simulink model "Simulator_3D2"  (R2018a)
settings: Solver=ode4  StartTime=0.0  StopTime=60  FixedStep=T  RelTol=1e-3
undefined symbols (not defined in the file): A_w, A_w2, epsilon_w, epsilon_w2, k_w, k_w2, Lc_0, omega_w, omega_w2, T, w_dir, w_dir2, zu_bar
libraries: vrlib x132
(part 6 of 6)

== system Simulator_3D2/Subsystem/5 static wave points7/Subsystem15/Subsystem ==
  note: Aw.Sin
  t : Inport
  x : Inport  Port=2
  Constant : Constant  Value=epsilon_w
  Gain : Gain  Gain=omega_w
  Gain1 : Gain  Gain=k_w
  Gain2 : Gain  Gain=A_w
  Gain5 : Gain  Gain=A_w*k_w
  Sum : Sum  Inputs=++-
  Trigonometric Function1 : Trigonometry  Operator=sincos
  Trigonometric Function2 : Trigonometry  Operator=atan
  direction : Gain  Gain=w_dir
  zeta(x,t) : Outport
  theta : Outport  Port=2
  wires:
  Trigonometric Function2/1 -> theta/1
  Gain5/1 -> Trigonometric Function2/1
  Trigonometric Function1/2 -> Gain5/1
  Gain/1 -> Sum/2
  Gain2/1 -> zeta(x,t)/1  "zeta(x,t)"
  Constant/1 -> Sum/1
  t/1 -> direction/1
  Gain1/1 -> Sum/3
  Trigonometric Function1/1 -> Gain2/1
  x/1 -> Gain1/1
  direction/1 -> Gain/1
  Sum/1 -> Trigonometric Function1/1

== system Simulator_3D2/Subsystem/5 static wave points7/Subsystem15/Subsystem1 ==
  note: Aw.Sin
  t : Inport
  x : Inport  Port=2
  Constant : Constant  Value=epsilon_w2
  Gain : Gain  Gain=omega_w2
  Gain1 : Gain  Gain=k_w2
  Gain2 : Gain  Gain=A_w2
  Gain5 : Gain  Gain=A_w2*k_w2
  Sum : Sum  Inputs=++-
  Trigonometric Function : Trigonometry  Operator=sincos
  Trigonometric Function1 : Trigonometry  Operator=atan
  direction : Gain  Gain=w_dir2
  zeta(x,t) : Outport
  theta : Outport  Port=2
  wires:
  Trigonometric Function/2 -> Gain5/1
  Trigonometric Function1/1 -> theta/1
  Gain5/1 -> Trigonometric Function1/1
  Sum/1 -> Trigonometric Function/1
  direction/1 -> Gain/1
  x/1 -> Gain1/1
  Trigonometric Function/1 -> Gain2/1
  Gain1/1 -> Sum/3
  t/1 -> direction/1
  Constant/1 -> Sum/1
  Gain2/1 -> zeta(x,t)/1  "zeta(x,t)"
  Gain/1 -> Sum/2

== system Simulator_3D2/Subsystem/5 static wave points7/Subsystem16/Subsystem ==
  note: Aw.Sin
  t : Inport
  x : Inport  Port=2
  Constant : Constant  Value=epsilon_w
  Gain : Gain  Gain=omega_w
  Gain1 : Gain  Gain=k_w
  Gain2 : Gain  Gain=A_w
  Gain5 : Gain  Gain=A_w*k_w
  Sum : Sum  Inputs=++-
  Trigonometric Function1 : Trigonometry  Operator=sincos
  Trigonometric Function2 : Trigonometry  Operator=atan
  direction : Gain  Gain=w_dir
  zeta(x,t) : Outport
  theta : Outport  Port=2
  wires:
  Sum/1 -> Trigonometric Function1/1
  direction/1 -> Gain/1
  x/1 -> Gain1/1
  Trigonometric Function1/1 -> Gain2/1
  Gain1/1 -> Sum/3
  t/1 -> direction/1
  Constant/1 -> Sum/1
  Gain2/1 -> zeta(x,t)/1  "zeta(x,t)"
  Gain/1 -> Sum/2
  Trigonometric Function1/2 -> Gain5/1
  Gain5/1 -> Trigonometric Function2/1
  Trigonometric Function2/1 -> theta/1

== system Simulator_3D2/Subsystem/5 static wave points7/Subsystem16/Subsystem1 ==
  note: Aw.Sin
  t : Inport
  x : Inport  Port=2
  Constant : Constant  Value=epsilon_w2
  Gain : Gain  Gain=omega_w2
  Gain1 : Gain  Gain=k_w2
  Gain2 : Gain  Gain=A_w2
  Gain5 : Gain  Gain=A_w2*k_w2
  Sum : Sum  Inputs=++-
  Trigonometric Function : Trigonometry  Operator=sincos
  Trigonometric Function1 : Trigonometry  Operator=atan
  direction : Gain  Gain=w_dir2
  zeta(x,t) : Outport
  theta : Outport  Port=2
  wires:
  Gain/1 -> Sum/2
  Gain2/1 -> zeta(x,t)/1  "zeta(x,t)"
  Constant/1 -> Sum/1
  t/1 -> direction/1
  Gain1/1 -> Sum/3
  Trigonometric Function/1 -> Gain2/1
  x/1 -> Gain1/1
  direction/1 -> Gain/1
  Sum/1 -> Trigonometric Function/1
  Gain5/1 -> Trigonometric Function1/1
  Trigonometric Function1/1 -> theta/1
  Trigonometric Function/2 -> Gain5/1

== system Simulator_3D2/Subsystem/followers/Subsystem1/Subsystem ==
  note: Aw.Sin
  t : Inport
  x : Inport  Port=2
  Constant : Constant  Value=epsilon_w
  Gain : Gain  Gain=omega_w
  Gain1 : Gain  Gain=k_w
  Gain2 : Gain  Gain=A_w
  Gain5 : Gain  Gain=A_w*k_w
  Sum : Sum  Inputs=++-
  Trigonometric Function1 : Trigonometry  Operator=sincos
  Trigonometric Function2 : Trigonometry  Operator=atan
  direction : Gain  Gain=w_dir
  zeta(x,t) : Outport
  theta : Outport  Port=2
  wires:
  Trigonometric Function2/1 -> theta/1
  Gain5/1 -> Trigonometric Function2/1
  Trigonometric Function1/2 -> Gain5/1
  Gain/1 -> Sum/2
  Gain2/1 -> zeta(x,t)/1  "zeta(x,t)"
  Constant/1 -> Sum/1
  t/1 -> direction/1
  Gain1/1 -> Sum/3
  Trigonometric Function1/1 -> Gain2/1
  x/1 -> Gain1/1
  direction/1 -> Gain/1
  Sum/1 -> Trigonometric Function1/1

== system Simulator_3D2/Subsystem/followers/Subsystem1/Subsystem1 ==
  note: Aw.Sin
  t : Inport
  x : Inport  Port=2
  Constant : Constant  Value=epsilon_w2
  Gain : Gain  Gain=omega_w2
  Gain1 : Gain  Gain=k_w2
  Gain2 : Gain  Gain=A_w2
  Gain5 : Gain  Gain=A_w2*k_w2
  Sum : Sum  Inputs=++-
  Trigonometric Function : Trigonometry  Operator=sincos
  Trigonometric Function1 : Trigonometry  Operator=atan
  direction : Gain  Gain=w_dir2
  zeta(x,t) : Outport
  theta : Outport  Port=2
  wires:
  Trigonometric Function/2 -> Gain5/1
  Trigonometric Function1/1 -> theta/1
  Gain5/1 -> Trigonometric Function1/1
  Sum/1 -> Trigonometric Function/1
  direction/1 -> Gain/1
  x/1 -> Gain1/1
  Trigonometric Function/1 -> Gain2/1
  Gain1/1 -> Sum/3
  t/1 -> direction/1
  Constant/1 -> Sum/1
  Gain2/1 -> zeta(x,t)/1  "zeta(x,t)"
  Gain/1 -> Sum/2

== system Simulator_3D2/Subsystem/followers/Subsystem2/Subsystem ==
  note: Aw.Sin
  t : Inport
  x : Inport  Port=2
  Constant : Constant  Value=epsilon_w
  Gain : Gain  Gain=omega_w
  Gain1 : Gain  Gain=k_w
  Gain2 : Gain  Gain=A_w
  Gain5 : Gain  Gain=A_w*k_w
  Sum : Sum  Inputs=++-
  Trigonometric Function1 : Trigonometry  Operator=sincos
  Trigonometric Function2 : Trigonometry  Operator=atan
  direction : Gain  Gain=w_dir
  zeta(x,t) : Outport
  theta : Outport  Port=2
  wires:
  Sum/1 -> Trigonometric Function1/1
  direction/1 -> Gain/1
  x/1 -> Gain1/1
  Trigonometric Function1/1 -> Gain2/1
  Gain1/1 -> Sum/3
  t/1 -> direction/1
  Constant/1 -> Sum/1
  Gain2/1 -> zeta(x,t)/1  "zeta(x,t)"
  Gain/1 -> Sum/2
  Trigonometric Function1/2 -> Gain5/1
  Gain5/1 -> Trigonometric Function2/1
  Trigonometric Function2/1 -> theta/1

== system Simulator_3D2/Subsystem/followers/Subsystem2/Subsystem1 ==
  note: Aw.Sin
  t : Inport
  x : Inport  Port=2
  Constant : Constant  Value=epsilon_w2
  Gain : Gain  Gain=omega_w2
  Gain1 : Gain  Gain=k_w2
  Gain2 : Gain  Gain=A_w2
  Gain5 : Gain  Gain=A_w2*k_w2
  Sum : Sum  Inputs=++-
  Trigonometric Function : Trigonometry  Operator=sincos
  Trigonometric Function1 : Trigonometry  Operator=atan
  direction : Gain  Gain=w_dir2
  zeta(x,t) : Outport
  theta : Outport  Port=2
  wires:
  Gain/1 -> Sum/2
  Gain2/1 -> zeta(x,t)/1  "zeta(x,t)"
  Constant/1 -> Sum/1
  t/1 -> direction/1
  Gain1/1 -> Sum/3
  Trigonometric Function/1 -> Gain2/1
  x/1 -> Gain1/1
  direction/1 -> Gain/1
  Sum/1 -> Trigonometric Function/1
  Gain5/1 -> Trigonometric Function1/1
  Trigonometric Function1/1 -> theta/1
  Trigonometric Function/2 -> Gain5/1

== system Simulator_3D2/Subsystem/followers/Subsystem3/Subsystem ==
  note: Aw.Sin
  t : Inport
  x : Inport  Port=2
  Constant : Constant  Value=epsilon_w
  Gain : Gain  Gain=omega_w
  Gain1 : Gain  Gain=k_w
  Gain2 : Gain  Gain=A_w
  Gain5 : Gain  Gain=A_w*k_w
  Sum : Sum  Inputs=++-
  Trigonometric Function1 : Trigonometry  Operator=sincos
  Trigonometric Function2 : Trigonometry  Operator=atan
  direction : Gain  Gain=w_dir
  zeta(x,t) : Outport
  theta : Outport  Port=2
  wires:
  Sum/1 -> Trigonometric Function1/1
  direction/1 -> Gain/1
  x/1 -> Gain1/1
  Trigonometric Function1/1 -> Gain2/1
  Gain1/1 -> Sum/3
  t/1 -> direction/1
  Constant/1 -> Sum/1
  Gain2/1 -> zeta(x,t)/1  "zeta(x,t)"
  Gain/1 -> Sum/2
  Trigonometric Function1/2 -> Gain5/1
  Gain5/1 -> Trigonometric Function2/1
  Trigonometric Function2/1 -> theta/1

== system Simulator_3D2/Subsystem/followers/Subsystem3/Subsystem1 ==
  note: Aw.Sin
  t : Inport
  x : Inport  Port=2
  Constant : Constant  Value=epsilon_w2
  Gain : Gain  Gain=omega_w2
  Gain1 : Gain  Gain=k_w2
  Gain2 : Gain  Gain=A_w2
  Gain5 : Gain  Gain=A_w2*k_w2
  Sum : Sum  Inputs=++-
  Trigonometric Function : Trigonometry  Operator=sincos
  Trigonometric Function1 : Trigonometry  Operator=atan
  direction : Gain  Gain=w_dir2
  zeta(x,t) : Outport
  theta : Outport  Port=2
  wires:
  Gain/1 -> Sum/2
  Gain2/1 -> zeta(x,t)/1  "zeta(x,t)"
  Constant/1 -> Sum/1
  t/1 -> direction/1
  Gain1/1 -> Sum/3
  Trigonometric Function/1 -> Gain2/1
  x/1 -> Gain1/1
  direction/1 -> Gain/1
  Sum/1 -> Trigonometric Function/1
  Gain5/1 -> Trigonometric Function1/1
  Trigonometric Function1/1 -> theta/1
  Trigonometric Function/2 -> Gain5/1

== system Simulator_3D2/Subsystem/followers/Subsystem4/Subsystem ==
  note: Aw.Sin
  t : Inport
  x : Inport  Port=2
  Constant : Constant  Value=epsilon_w
  Gain : Gain  Gain=omega_w
  Gain1 : Gain  Gain=k_w
  Gain2 : Gain  Gain=A_w
  Gain5 : Gain  Gain=A_w*k_w
  Sum : Sum  Inputs=++-
  Trigonometric Function1 : Trigonometry  Operator=sincos
  Trigonometric Function2 : Trigonometry  Operator=atan
  direction : Gain  Gain=w_dir
  zeta(x,t) : Outport
  theta : Outport  Port=2
  wires:
  Trigonometric Function2/1 -> theta/1
  Gain5/1 -> Trigonometric Function2/1
  Trigonometric Function1/2 -> Gain5/1
  Gain/1 -> Sum/2
  Gain2/1 -> zeta(x,t)/1  "zeta(x,t)"
  Constant/1 -> Sum/1
  t/1 -> direction/1
  Gain1/1 -> Sum/3
  Trigonometric Function1/1 -> Gain2/1
  x/1 -> Gain1/1
  direction/1 -> Gain/1
  Sum/1 -> Trigonometric Function1/1

== system Simulator_3D2/Subsystem/followers/Subsystem4/Subsystem1 ==
  note: Aw.Sin
  t : Inport
  x : Inport  Port=2
  Constant : Constant  Value=epsilon_w2
  Gain : Gain  Gain=omega_w2
  Gain1 : Gain  Gain=k_w2
  Gain2 : Gain  Gain=A_w2
  Gain5 : Gain  Gain=A_w2*k_w2
  Sum : Sum  Inputs=++-
  Trigonometric Function : Trigonometry  Operator=sincos
  Trigonometric Function1 : Trigonometry  Operator=atan
  direction : Gain  Gain=w_dir2
  zeta(x,t) : Outport
  theta : Outport  Port=2
  wires:
  Trigonometric Function/2 -> Gain5/1
  Trigonometric Function1/1 -> theta/1
  Gain5/1 -> Trigonometric Function1/1
  Sum/1 -> Trigonometric Function/1
  direction/1 -> Gain/1
  x/1 -> Gain1/1
  Trigonometric Function/1 -> Gain2/1
  Gain1/1 -> Sum/3
  t/1 -> direction/1
  Constant/1 -> Sum/1
  Gain2/1 -> zeta(x,t)/1  "zeta(x,t)"
  Gain/1 -> Sum/2

== system Simulator_3D2/Subsystem/followers/Subsystem5/Subsystem ==
  note: Aw.Sin
  t : Inport
  x : Inport  Port=2
  Constant : Constant  Value=epsilon_w
  Gain : Gain  Gain=omega_w
  Gain1 : Gain  Gain=k_w
  Gain2 : Gain  Gain=A_w
  Gain5 : Gain  Gain=A_w*k_w
  Sum : Sum  Inputs=++-
  Trigonometric Function1 : Trigonometry  Operator=sincos
  Trigonometric Function2 : Trigonometry  Operator=atan
  direction : Gain  Gain=w_dir
  zeta(x,t) : Outport
  theta : Outport  Port=2
  wires:
  Sum/1 -> Trigonometric Function1/1
  direction/1 -> Gain/1
  x/1 -> Gain1/1
  Trigonometric Function1/1 -> Gain2/1
  Gain1/1 -> Sum/3
  t/1 -> direction/1
  Constant/1 -> Sum/1
  Gain2/1 -> zeta(x,t)/1  "zeta(x,t)"
  Gain/1 -> Sum/2
  Trigonometric Function1/2 -> Gain5/1
  Gain5/1 -> Trigonometric Function2/1
  Trigonometric Function2/1 -> theta/1

== system Simulator_3D2/Subsystem/followers/Subsystem5/Subsystem1 ==
  note: Aw.Sin
  t : Inport
  x : Inport  Port=2
  Constant : Constant  Value=epsilon_w2
  Gain : Gain  Gain=omega_w2
  Gain1 : Gain  Gain=k_w2
  Gain2 : Gain  Gain=A_w2
  Gain5 : Gain  Gain=A_w2*k_w2
  Sum : Sum  Inputs=++-
  Trigonometric Function : Trigonometry  Operator=sincos
  Trigonometric Function1 : Trigonometry  Operator=atan
  direction : Gain  Gain=w_dir2
  zeta(x,t) : Outport
  theta : Outport  Port=2
  wires:
  Gain/1 -> Sum/2
  Gain2/1 -> zeta(x,t)/1  "zeta(x,t)"
  Constant/1 -> Sum/1
  t/1 -> direction/1
  Gain1/1 -> Sum/3
  Trigonometric Function/1 -> Gain2/1
  x/1 -> Gain1/1
  direction/1 -> Gain/1
  Sum/1 -> Trigonometric Function/1
  Gain5/1 -> Trigonometric Function1/1
  Trigonometric Function1/1 -> theta/1
  Trigonometric Function/2 -> Gain5/1

== system Simulator_3D2/Subsystem/followers/Subsystem6/Subsystem ==
  note: Aw.Sin
  t : Inport
  x : Inport  Port=2
  Constant : Constant  Value=epsilon_w
  Gain : Gain  Gain=omega_w
  Gain1 : Gain  Gain=k_w
  Gain2 : Gain  Gain=A_w
  Gain5 : Gain  Gain=A_w*k_w
  Sum : Sum  Inputs=++-
  Trigonometric Function1 : Trigonometry  Operator=sincos
  Trigonometric Function2 : Trigonometry  Operator=atan
  direction : Gain  Gain=w_dir
  zeta(x,t) : Outport
  theta : Outport  Port=2
  wires:
  Trigonometric Function2/1 -> theta/1
  Gain5/1 -> Trigonometric Function2/1
  Trigonometric Function1/2 -> Gain5/1
  Gain/1 -> Sum/2
  Gain2/1 -> zeta(x,t)/1  "zeta(x,t)"
  Constant/1 -> Sum/1
  t/1 -> direction/1
  Gain1/1 -> Sum/3
  Trigonometric Function1/1 -> Gain2/1
  x/1 -> Gain1/1
  direction/1 -> Gain/1
  Sum/1 -> Trigonometric Function1/1

== system Simulator_3D2/Subsystem/followers/Subsystem6/Subsystem1 ==
  note: Aw.Sin
  t : Inport
  x : Inport  Port=2
  Constant : Constant  Value=epsilon_w2
  Gain : Gain  Gain=omega_w2
  Gain1 : Gain  Gain=k_w2
  Gain2 : Gain  Gain=A_w2
  Gain5 : Gain  Gain=A_w2*k_w2
  Sum : Sum  Inputs=++-
  Trigonometric Function : Trigonometry  Operator=sincos
  Trigonometric Function1 : Trigonometry  Operator=atan
  direction : Gain  Gain=w_dir2
  zeta(x,t) : Outport
  theta : Outport  Port=2
  wires:
  Trigonometric Function/2 -> Gain5/1
  Trigonometric Function1/1 -> theta/1
  Gain5/1 -> Trigonometric Function1/1
  Sum/1 -> Trigonometric Function/1
  direction/1 -> Gain/1
  x/1 -> Gain1/1
  Trigonometric Function/1 -> Gain2/1
  Gain1/1 -> Sum/3
  t/1 -> direction/1
  Constant/1 -> Sum/1
  Gain2/1 -> zeta(x,t)/1  "zeta(x,t)"
  Gain/1 -> Sum/2

== system Simulator_3D2/Subsystem/followers/Subsystem7/Subsystem ==
  note: Aw.Sin
  t : Inport
  x : Inport  Port=2
  Constant : Constant  Value=epsilon_w
  Gain : Gain  Gain=omega_w
  Gain1 : Gain  Gain=k_w
  Gain2 : Gain  Gain=A_w
  Gain5 : Gain  Gain=A_w*k_w
  Sum : Sum  Inputs=++-
  Trigonometric Function1 : Trigonometry  Operator=sincos
  Trigonometric Function2 : Trigonometry  Operator=atan
  direction : Gain  Gain=w_dir
  zeta(x,t) : Outport
  theta : Outport  Port=2
  wires:
  Sum/1 -> Trigonometric Function1/1
  direction/1 -> Gain/1
  x/1 -> Gain1/1
  Trigonometric Function1/1 -> Gain2/1
  Gain1/1 -> Sum/3
  t/1 -> direction/1
  Constant/1 -> Sum/1
  Gain2/1 -> zeta(x,t)/1  "zeta(x,t)"
  Gain/1 -> Sum/2
  Trigonometric Function1/2 -> Gain5/1
  Gain5/1 -> Trigonometric Function2/1
  Trigonometric Function2/1 -> theta/1

== system Simulator_3D2/Subsystem/followers/Subsystem7/Subsystem1 ==
  note: Aw.Sin
  t : Inport
  x : Inport  Port=2
  Constant : Constant  Value=epsilon_w2
  Gain : Gain  Gain=omega_w2
  Gain1 : Gain  Gain=k_w2
  Gain2 : Gain  Gain=A_w2
  Gain5 : Gain  Gain=A_w2*k_w2
  Sum : Sum  Inputs=++-
  Trigonometric Function : Trigonometry  Operator=sincos
  Trigonometric Function1 : Trigonometry  Operator=atan
  direction : Gain  Gain=w_dir2
  zeta(x,t) : Outport
  theta : Outport  Port=2
  wires:
  Gain/1 -> Sum/2
  Gain2/1 -> zeta(x,t)/1  "zeta(x,t)"
  Constant/1 -> Sum/1
  t/1 -> direction/1
  Gain1/1 -> Sum/3
  Trigonometric Function/1 -> Gain2/1
  x/1 -> Gain1/1
  direction/1 -> Gain/1
  Sum/1 -> Trigonometric Function/1
  Gain5/1 -> Trigonometric Function1/1
  Trigonometric Function1/1 -> theta/1
  Trigonometric Function/2 -> Gain5/1

== system Simulator_3D2/Subsystem/followers/Subsystem8/Subsystem ==
  note: Aw.Sin
  t : Inport
  x : Inport  Port=2
  Constant : Constant  Value=epsilon_w
  Gain : Gain  Gain=omega_w
  Gain1 : Gain  Gain=k_w
  Gain2 : Gain  Gain=A_w
  Gain5 : Gain  Gain=A_w*k_w
  Sum : Sum  Inputs=++-
  Trigonometric Function1 : Trigonometry  Operator=sincos
  Trigonometric Function2 : Trigonometry  Operator=atan
  direction : Gain  Gain=w_dir
  zeta(x,t) : Outport
  theta : Outport  Port=2
  wires:
  Trigonometric Function2/1 -> theta/1
  Gain5/1 -> Trigonometric Function2/1
  Trigonometric Function1/2 -> Gain5/1
  Gain/1 -> Sum/2
  Gain2/1 -> zeta(x,t)/1  "zeta(x,t)"
  Constant/1 -> Sum/1
  t/1 -> direction/1
  Gain1/1 -> Sum/3
  Trigonometric Function1/1 -> Gain2/1
  x/1 -> Gain1/1
  direction/1 -> Gain/1
  Sum/1 -> Trigonometric Function1/1

== system Simulator_3D2/Subsystem/followers/Subsystem8/Subsystem1 ==
  note: Aw.Sin
  t : Inport
  x : Inport  Port=2
  Constant : Constant  Value=epsilon_w2
  Gain : Gain  Gain=omega_w2
  Gain1 : Gain  Gain=k_w2
  Gain2 : Gain  Gain=A_w2
  Gain5 : Gain  Gain=A_w2*k_w2
  Sum : Sum  Inputs=++-
  Trigonometric Function : Trigonometry  Operator=sincos
  Trigonometric Function1 : Trigonometry  Operator=atan
  direction : Gain  Gain=w_dir2
  zeta(x,t) : Outport
  theta : Outport  Port=2
  wires:
  Trigonometric Function/2 -> Gain5/1
  Trigonometric Function1/1 -> theta/1
  Gain5/1 -> Trigonometric Function1/1
  Sum/1 -> Trigonometric Function/1
  direction/1 -> Gain/1
  x/1 -> Gain1/1
  Trigonometric Function/1 -> Gain2/1
  Gain1/1 -> Sum/3
  t/1 -> direction/1
  Constant/1 -> Sum/1
  Gain2/1 -> zeta(x,t)/1  "zeta(x,t)"
  Gain/1 -> Sum/2
